simulink model "video1"  (R2020a)
settings: Solver=FixedStepDiscrete  StartTime=0.0  StopTime=10.0  FixedStep=0.01  RelTol=1e-3
undefined symbols (not defined in the file or in its folder): ticksPerRot, wheelR
libraries: mobileRoboticsTrainingLib x5
settings Model: Creator=Navyasree  LastModifiedBy=Navyasree

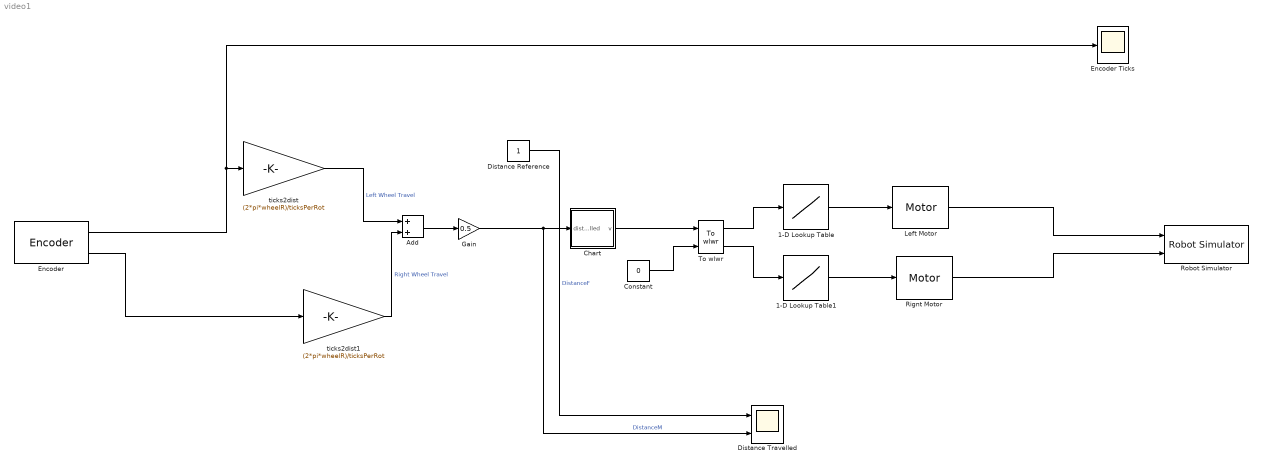
== system video1 ==
  1-D Lookup Table : Lookup_n-D  NumberOfTableDimensions=1  BreakpointsForDimension1=[-5:5]  Table=tanh([-5:5])  InternalRulePriority=Speed  RndMeth=Simplest  InputSameDT=on
  1-D Lookup Table1 : Lookup_n-D  NumberOfTableDimensions=1  BreakpointsForDimension1=[-5:5]  Table=tanh([-5:5])  InternalRulePriority=Speed  RndMeth=Simplest  InputSameDT=on
  Add : Sum
  Chart : Stateflow chart  TreatAsAtomicUnit=on
  Constant : Constant  Value=0
  Distance Reference : Constant
  Distance Travelled : Scope  NumInputPorts=2
  Encoder : mobileRoboticsTrainingLib/Encoder  axleLength=axleLength  wheelR=wheelR  ticksPerRot=ticksPerRot
      settings: SourceProductName=Mobile Robotics Training Library
  Encoder Ticks : Scope
  Gain : Gain  Gain=0.5
  Left Motor : mobileRoboticsTrainingLib/Motor  motorPlant=wheelR  sensorType=Speed
      settings: SourceProductName=Mobile Robotics Training Library
  Rignt Motor : mobileRoboticsTrainingLib/Motor  motorPlant=wheelR  sensorType=Speed
      settings: SourceProductName=Mobile Robotics Training Library
  Robot Simulator : mobileRoboticsTrainingLib/Robot Simulator  Priority=99  mapVar=[]  startX=1  startY=1  startTheta=0  axleLength=0.1  wheelR=0.05
  To wlwr : mobileRoboticsTrainingLib/To wlwr  axleLength=axleLength  wheelR=wheelR
  ticks2dist : Gain  Gain=(2*pi*wheelR)/ticksPerRot
  ticks2dist1 : Gain  Gain=(2*pi*wheelR)/ticksPerRot
  wires:
  ticks2dist/1 -> Add/1  "Left Wheel Travel"
  Encoder/1 -> Encoder Ticks/1, ticks2dist/1
  Encoder/2 -> ticks2dist1/1
  ticks2dist1/1 -> Add/2  "Right Wheel Travel"
  Gain/1 -> Distance Travelled/2, Chart/1(distTravelled)  "DistanceM"
  Add/1 -> Gain/1
  Chart/1(v) -> To wlwr/1
  Distance Reference/1 -> Distance Travelled/1  "DistanceF"
  To wlwr/1 -> 1-D Lookup Table/1
  To wlwr/2 -> 1-D Lookup Table1/1
  Constant/1 -> To wlwr/2
  1-D Lookup Table/1 -> Left Motor/1
  1-D Lookup Table1/1 -> Rignt Motor/1
  Left Motor/1 -> Robot Simulator/1
  Rignt Motor/1 -> Robot Simulator/2

== stateflow chart video1/Chart ==
  state MoveForward
    entry:v = 0.1
  state Stop
    entry:v= 0
  (default) -> MoveForward
  MoveForward -> Stop : [distTravelled>=1]
  data: distTravelled input; v output
